simulink model "quadtank"  (Simulink 7.7)
settings: Solver=ode23  StartTime=0.0  StopTime=40  FixedStep=1  RelTol=1e-3
PreLoadFcn:
  | ref_option=0
  | initialize
values from neighbouring files (symbols this model uses):
  mpc_prob = rmfield(mpc_prob,d(fields))    [compute_coupling.m]    (also in tankGUI.m = evalin('base','mpc_prob'); tankinformation.m = compute_coupling(mpc_prob,A,B))
settings Model: Creator=root  LastModifiedBy=root  BufferReuse=off
settings SolverCC: AutoInsertRateTranBlk=on
settings DataIOCC: ExternalInput=model_bus
settings OptimizationCC: OptimizeBlockIOStorage=off  BufferReuse=off  ExpressionFolding=off  LocalBlockOutputs=off
settings DebuggingCC: StrictBusMsg=Warning
settings SFSimCC: SimParseCustomCode=off

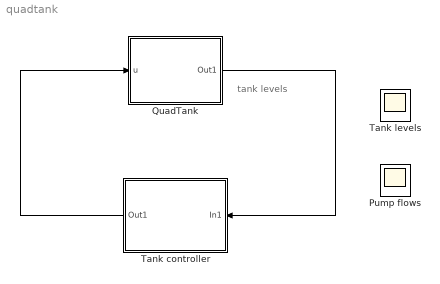
== system quadtank ==
  note: tank levels
  Pump flows : Scope  NumInputPorts=2
      settings: Floating=on  YMin=0~0  YMax=0.6~0.6
  QuadTank : Subsystem
      mask Display: disp('Quadtank');
  Tank controller : Subsystem  RequirementInfo="{}  %GIDa_28b16a57_7a0b_4540_a2f5_635bf4650807"
      mask Display: disp('Controller');
  Tank levels : Scope  NumInputPorts=4
      settings: Floating=on  YMin=0~0~0~0  YMax=0.6~0.6~0.6~0.6  SampleInput=on
  wires:
  QuadTank/1(Out1) -> Tank controller/1(In1)
  Tank controller/1(Out1) -> QuadTank/1(u)

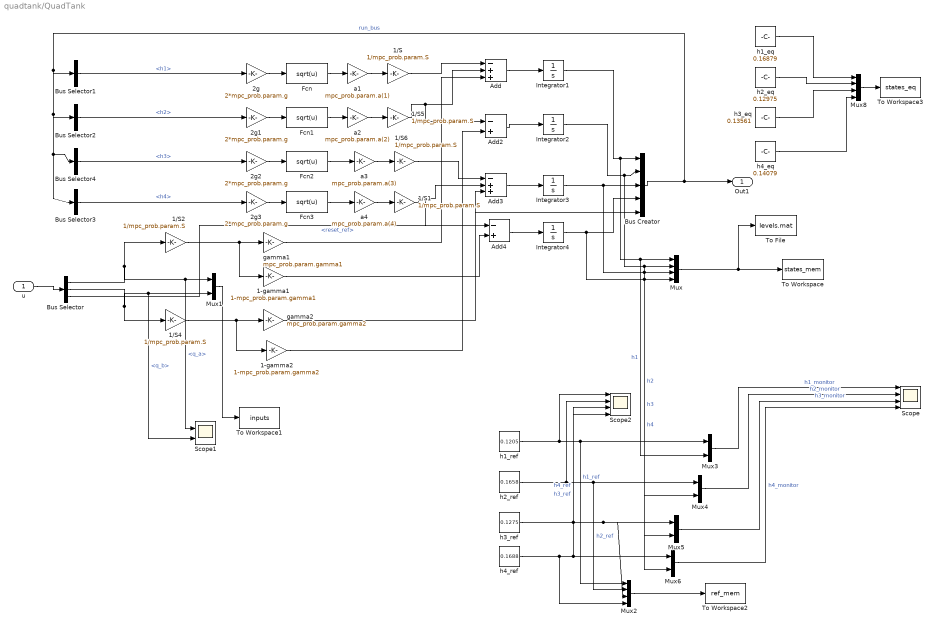
== system quadtank/QuadTank ==
  u : Inport
  1-gamma1 : Gain  Gain=1-mpc_prob.param.gamma1
  1-gamma2 : Gain  Gain=1-mpc_prob.param.gamma2
  1/S{,1..2,4..6} (6 alike) : Gain  Gain=1/mpc_prob.param.S
  2g{,1..3} (4 alike) : Gain  Gain=2*mpc_prob.param.g
  Add : Sum  Inputs=-++
  Add2 : Sum  Inputs=-+
  Add3 : Sum  Inputs=-++
  Add4 : Sum  Inputs=-+
  Bus Creator : BusCreator  Inputs='h1','h2','h3','h4','reset_ref'  OutDataTypeStr=Bus: run_bus
  Bus Selector : BusSelector  OutputSignals=q_a,q_b,reset_ref
  Bus Selector1 : BusSelector  OutputSignals=h1
  Bus Selector2 : BusSelector  OutputSignals=h2
  Bus Selector3 : BusSelector  OutputSignals=h4
  Bus Selector4 : BusSelector  OutputSignals=h3
  Fcn{,1..3} (4 alike) : Fcn  Expr=sqrt(u)
  Integrator1 : Integrator  InitialCondition=mpc_prob.init.h1
  Integrator2 : Integrator  InitialCondition=mpc_prob.init.h2
  Integrator3 : Integrator  InitialCondition=mpc_prob.init.h3
  Integrator4 : Integrator  InitialCondition=mpc_prob.init.h4
  Mux : Mux
  Mux{1,3..6} (5 alike) : Mux  Inputs=2
  Mux2 : Mux
  Mux8 : Mux
  Scope : Scope  NumInputPorts=4
      settings: TimeRange=0.45  YMin=0.565~0.325~0.05~0.54  YMax=0.61~0.6~0.6~0.6  SaveName=ScopeData2
  Scope1 : Scope  NumInputPorts=2
      settings: YMin=-5~-5  YMax=5~5  SaveName=ScopeData3
  Scope2 : Scope  NumInputPorts=4
      settings: TimeRange=1  YMin=0.2~0.15~0.1~0.15  YMax=0.3~0.5~0.4~0.5  SaveName=ScopeData7
  To File : ToFile  Filename=levels.mat
  To Workspace : ToWorkspace  VariableName=states_mem  SampleTime=-1  SaveFormat=Array
  To Workspace1 : ToWorkspace  VariableName=inputs  SampleTime=-1  SaveFormat=Array
  To Workspace2 : ToWorkspace  VariableName=ref_mem  SampleTime=-1  SaveFormat=Array
  To Workspace3 : ToWorkspace  VariableName=states_eq  SampleTime=-1  SaveFormat=Array
  a1 : Gain  Gain=mpc_prob.param.a(1)
  a2 : Gain  Gain=mpc_prob.param.a(2)
  a3 : Gain  Gain=mpc_prob.param.a(3)
  a4 : Gain  Gain=mpc_prob.param.a(4)
  gamma1 : Gain  Gain=mpc_prob.param.gamma1
  gamma2 : Gain  Gain=mpc_prob.param.gamma2
  h1_eq : Constant  Value=0.16879  VectorParams1D=off
  h1_ref : Constant  Value=0.1205  VectorParams1D=off
  h2_eq : Constant  Value=0.12975  VectorParams1D=off
  h2_ref : Constant  Value=0.1658  VectorParams1D=off
  h3_eq : Constant  Value=0.13561  VectorParams1D=off
  h3_ref : Constant  Value=0.1275  VectorParams1D=off
  h4_eq : Constant  Value=0.14079  VectorParams1D=off
  h4_ref : Constant  Value=0.1688  VectorParams1D=off
  Out1 : Outport
  wires:
  2g/1 -> Fcn/1
  2g1/1 -> Fcn1/1
  2g2/1 -> Fcn2/1
  2g3/1 -> Fcn3/1
  Fcn/1 -> a1/1
  a1/1 -> 1/S/1
  Fcn3/1 -> a4/1
  a4/1 -> 1/S1/1
  Fcn1/1 -> a2/1
  Fcn2/1 -> a3/1
  a2/1 -> 1/S5/1
  a3/1 -> 1/S6/1
  u/1 -> Bus Selector/1
  Add/1 -> Integrator1/1
  Add2/1 -> Integrator2/1
  Add3/1 -> Integrator3/1
  Add4/1 -> Integrator4/1
  Bus Selector/1 -> 1/S2/1, Mux1/1, Scope1/1  "<q_a>"
  Bus Selector/2 -> 1/S4/1, Mux1/2, Scope1/2  "<q_b>"
  1/S2/1 -> gamma1/1, 1-gamma1/1
  1/S4/1 -> gamma2/1, 1-gamma2/1
  Bus Creator/1 -> Out1/1, Bus Selector1/1, Bus Selector2/1, Bus Selector4/1, Bus Selector3/1  "run_bus"
  Bus Selector1/1 -> 2g/1  "<h1>"
  Bus Selector2/1 -> 2g1/1  "<h2>"
  Bus Selector4/1 -> 2g2/1  "<h3>"
  Bus Selector3/1 -> 2g3/1  "<h4>"
  Integrator1/1 -> Bus Creator/1, Mux/1, Mux3/2  "h1"
  Integrator2/1 -> Bus Creator/2, Mux/2, Mux4/2  "h2"
  Integrator3/1 -> Bus Creator/3, Mux/3, Mux5/2  "h3"
  Integrator4/1 -> Bus Creator/4, Mux/4, Mux6/2  "h4"
  Mux/1 -> To Workspace/1, To File/1
  h1_ref/1 -> Mux3/1, Mux2/1, Scope2/1  "h1_ref"
  h2_ref/1 -> Mux4/1, Mux2/2, Scope2/2  "h2_ref"
  h3_ref/1 -> Mux5/1, Mux2/3, Scope2/3  "h3_ref"
  h4_ref/1 -> Mux2/4, Mux6/1, Scope2/4  "h4_ref"
  Mux3/1 -> Scope/1  "h1_monitor"
  Mux4/1 -> Scope/2  "h2_monitor"
  Mux5/1 -> Scope/3  "h3_monitor"
  Mux6/1 -> Scope/4  "h4_monitor"
  1/S/1 -> Add/1
  1/S5/1 -> Add/2, Add2/1
  gamma1/1 -> Add/3
  1-gamma2/1 -> Add2/2
  1/S6/1 -> Add3/1
  1/S1/1 -> Add3/2, Add4/1
  gamma2/1 -> Add3/3
  1-gamma1/1 -> Add4/2
  Bus Selector/3 -> Bus Creator/5  "<reset_ref>"
  Mux2/1 -> To Workspace2/1
  h1_eq/1 -> Mux8/1
  h2_eq/1 -> Mux8/2
  h3_eq/1 -> Mux8/3
  h4_eq/1 -> Mux8/4
  Mux8/1 -> To Workspace3/1
  Mux1/1 -> To Workspace1/1

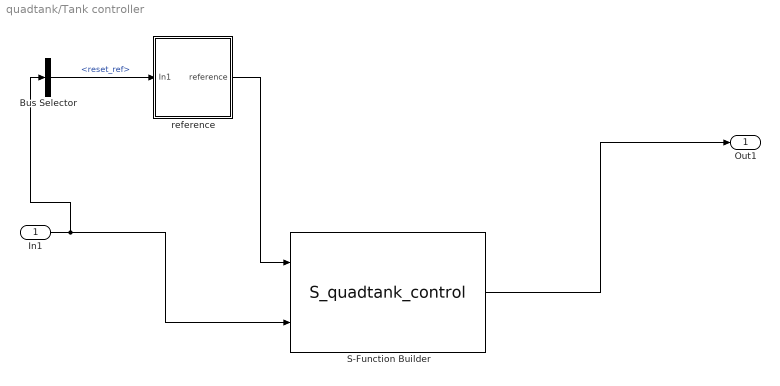
== system quadtank/Tank controller ==
  In1 : Inport
  Bus Selector : BusSelector  OutputSignals=reset_ref
  S-Function Builder : S-Function  InitFcn=try, set_param(gcb,'FunctionName','S_quadtank_control'), end  FunctionName=S_quadtank_control  SFunctionModules=S_quadtank_control_wrapper  WizardData=DataTag0  EnableBusSupport=off  mask(S-Function Builder){}
      mask help: The S-Function Builder block creates a wrapper C-MEX S-function from your supplied C code with multiple input ports, output ports, and a variable number of scalar, vector, or matrix parameters. The input and output ports can propagate Simulink built-in data types, fixed-point datatypes, complex, frame, 1-D, and 2-D signals. This block also supports discrete and continuous states of type real. You can optionally have the block generate a TLC file to be used with Real-Time Workshop for code generation.
      mask init:
      | val = [[.9  0.75 0.75 1 1 .9 .9 1]',[1 1 0.75 0.75 .9 .9 1 .9]'];try , sys = get_param(gcb,'SfunBuilderFcnName');if isempty(sys), sys = get_param(gcb,'FunctionName'); end,catch, sys = get_param(gcb,'FunctionName'); end
      settings: CopyFcn=set_param(gcbh,'LinkStatus','none')  PreSaveFcn=try, set_param(gcb,'FunctionName','S_quadtank_control'), end  OpenFcn=sfunctionwizard(gcbh)
      mask Display:
      | plot(val(:,1),val(:,2)),disp(sys)
      | port_label('input',1,'ref')
      | port_label('input',2,'x')
      | port_label('output',1,'u')
  reference : Subsystem
  Out1 : Outport
  wires:
  reference/1(reference) -> S-Function Builder/1
  In1/1 -> S-Function Builder/2, Bus Selector/1
  S-Function Builder/1 -> Out1/1
  Bus Selector/1 -> reference/1(In1)  "<reset_ref>"

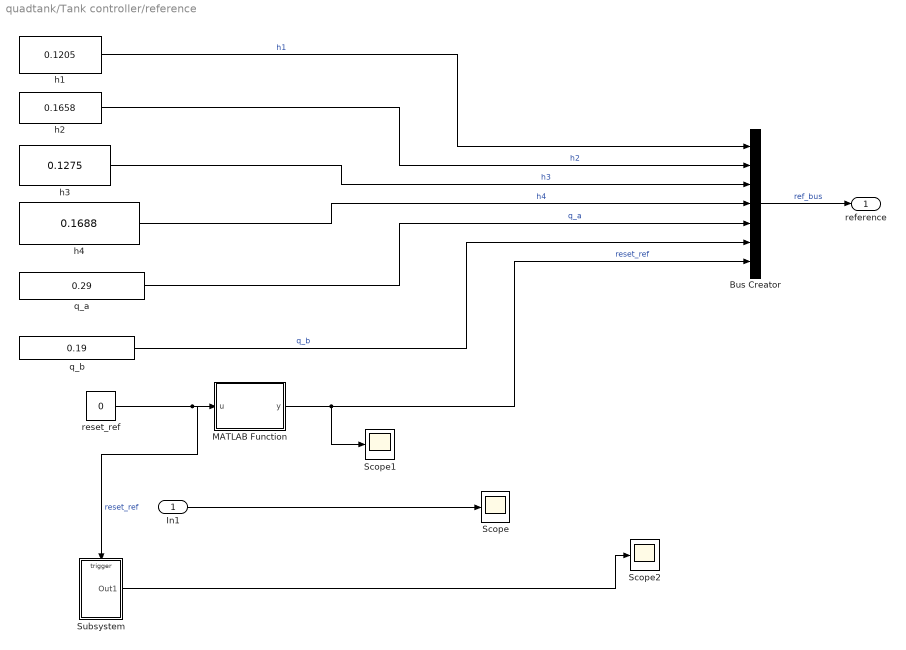
== system quadtank/Tank controller/reference ==
  In1 : Inport
  Bus Creator : BusCreator  Inputs=7  OutDataTypeStr=Bus: ref_bus
  MATLAB Function : Stateflow chart  TreatAsAtomicUnit=on
  Scope : Scope
      settings: SaveName=ScopeData5
  Scope1 : Scope
      settings: SaveName=ScopeData4
  Scope2 : Scope
      settings: SaveName=ScopeData6
  Subsystem : Subsystem
  h1 : Constant  Value=0.1205  VectorParams1D=off
  h2 : Constant  Value=0.1658  VectorParams1D=off
  h3 : Constant  Value=0.1275  VectorParams1D=off
  h4 : Constant  Value=0.1688  VectorParams1D=off
  q_a : Constant  Value=0.29  VectorParams1D=off
  q_b : Constant  Value=0.19  VectorParams1D=off
  reset_ref : Constant  Value=0
  reference : Outport
  wires:
  Bus Creator/1 -> reference/1  "ref_bus"
  h1/1 -> Bus Creator/1  "h1"
  h2/1 -> Bus Creator/2  "h2"
  h3/1 -> Bus Creator/3  "h3"
  h4/1 -> Bus Creator/4  "h4"
  q_a/1 -> Bus Creator/5  "q_a"
  q_b/1 -> Bus Creator/6  "q_b"
  In1/1 -> Scope/1
  reset_ref/1 -> MATLAB Function/1(u), Subsystem/Trigger  "reset_ref"
  MATLAB Function/1(y) -> Bus Creator/7, Scope1/1  "reset_ref"
  Subsystem/1(Out1) -> Scope2/1

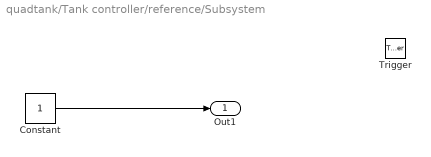
== system quadtank/Tank controller/reference/Subsystem ==
  Trigger : TriggerPort
  Constant : Constant
  Out1 : Outport
  wires:
  Constant/1 -> Out1/1

== matlab function Tank controller/reference/MATLAB Function ==
  data: u input double; y output double
function y=fcn(u)
%#codegen
eml.extrinsic('set_param');
eml.extrinsic('num2str');

if(u==1)
set_param('quadtank/Tank controller/reference/reset_ref','Value',num2str(0));
y=u;
else
    y=u;
end
